simulink model "Kimura_simulink"  (R2022b)
settings: Solver=ode45  StartTime=0.0  StopTime=10  RelTol=1e-3  AbsTol=1e-6
settings Model: Creator=MSC Software  LastModifiedBy=Administrator
settings SolverCC: AutoScaleAbsTol=off  AlgebraicLoopSolver=TrustRegion
settings DataIOCC: SaveFormat=Array  SignalLoggingSaveFormat=ModelDataLogs  ReturnWorkspaceOutputs=off
settings OptimizationCC: BlockReduction=off  BooleanDataType=off  ExpressionDepthLimit=2147483647  InitFltsAndDblsToZero=on  LifeSpan=inf
settings DebuggingCC: SaveWithParameterizedLinksMsg=none  UnderspecifiedInitializationDetection=Classic  MergeDetectMultiDrivingBlocksExec=none  SignalResolutionControl=TryResolveAllWithWarning  MultiTaskDSMMsg=warning  MultiTaskCondExecSysMsg=none  FcnCallInpInsideContextMsg=warning  UnconnectedInputMsg=warning  UnconnectedOutputMsg=warning  UnconnectedLineMsg=warning  StateNameClashWarn=warning  SFUnexpectedBacktrackingDiag=warning  SFNoUnconditionalDefaultTransitionDiag=warning  SFExecutionAtInitializationDiag=none  SFMachineParentedDataDiag=warning  ArithmeticOperatorsInVariantConditions=warning
settings HardwareCC: ProdBitPerPointer=32  ProdBitPerSizeT=32  ProdBitPerPtrDiffT=32  ProdLargestAtomicFloat=None  ProdIntDivRoundTo=Undefined  ProdEndianess=Unspecified  ProdWordSize=32  ProdHWDeviceType=32-bit Generic  TargetUnknown=on
settings ModelReferenceCC: EnableRefExpFcnMdlSchedulingChecks=on  PropagateSignalLabelsOutOfModel=off
settings SFSimCC: SimUseLocalCustomCode=off  CustomCodeUndefinedFunction=UseInterfaceOnly
settings RTWCC: TemplateMakefile=grt_unix.tmf  RTWUseLocalCustomCode=off
settings CodeAppCC: StateflowObjectComments=on
settings GRTTargetCC: TargetFcnLib=ansi_tfl_tmw.mat  TargetLangStandard=C89/C90 (ANSI)  CombineOutputUpdateFcns=off  GRTInterface=on
settings ConfigComp: CovMetricSettings=dw  CovSaveCumulativeToWorkspaceVar=on  CovSaveSingleToWorkspaceVar=on  CovExternalEMLEnable=off

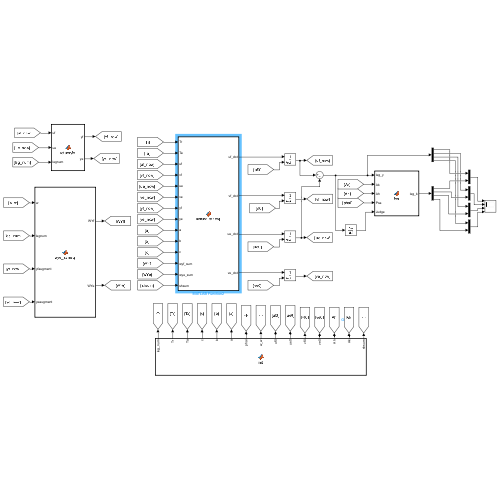
[thumbnail: Simulink's stored preview of the top-level diagram]
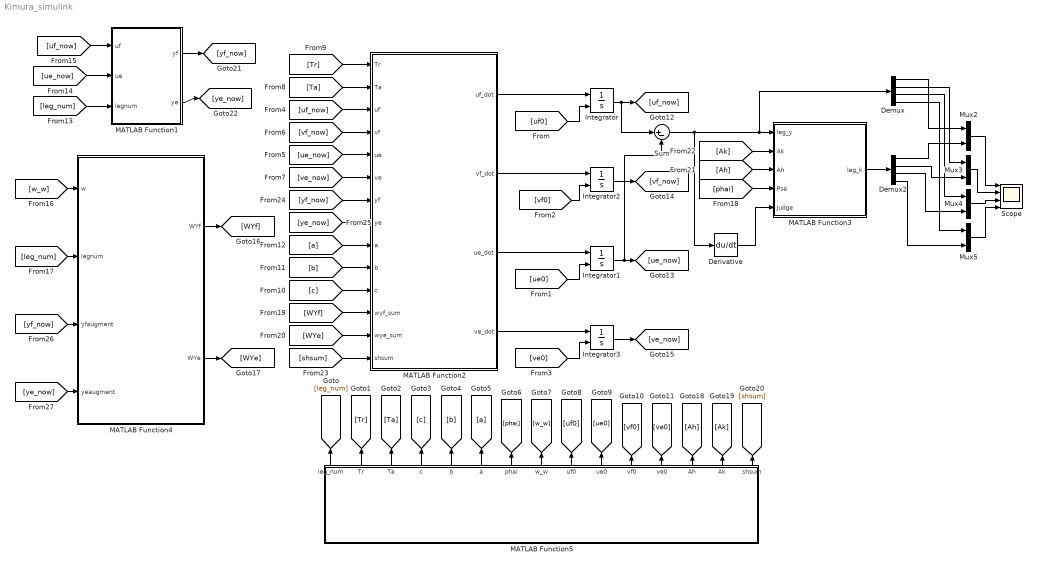
== system Kimura_simulink ==
  Demux : Demux
  Demux2 : Demux
  Derivative : Derivative
  Integrator{,1..3} (4 alike) : Integrator  InitialConditionSource=external
  MATLAB Function1 : MATLAB Function  TreatAsAtomicUnit=on
  MATLAB Function2 : MATLAB Function  TreatAsAtomicUnit=on
  MATLAB Function3 : MATLAB Function  TreatAsAtomicUnit=on
  MATLAB Function4 : MATLAB Function  TreatAsAtomicUnit=on
  MATLAB Function5 : MATLAB Function  TreatAsAtomicUnit=on
  Mux{2..5} (4 alike) : Mux  Inputs=2
  Scope : Scope  NumInputPorts=4
  Sum : Sum  Inputs=|+-
  wires:
  MATLAB Function2/4(ve_dot) -> Integrator3/1
  Demux/1 -> Mux2/1
  Mux5/1 -> Scope/4
  Demux/2 -> Mux3/1
  Demux/3 -> Mux4/1
  Mux4/1 -> Scope/3
  Demux2/3 -> Mux4/2
  Demux2/4 -> Mux5/2
  Demux2/1 -> Mux2/2
  Mux2/1 -> Scope/1
  Mux3/1 -> Scope/2
  MATLAB Function2/1(uf_dot) -> Integrator/1
  Demux2/2 -> Mux3/2
  Demux/4 -> Mux5/1
  MATLAB Function3/1(leg_k) -> Demux2/1
  MATLAB Function5/1(leg_num) -> [leg_num]
  MATLAB Function5/2(Tr) -> [Tr]
  MATLAB Function5/3(Ta) -> [Ta]
  MATLAB Function5/4(c) -> [c]
  MATLAB Function5/5(b) -> [b]
  MATLAB Function5/6(a) -> [a]
  MATLAB Function5/7(phai) -> [phai]
  MATLAB Function5/8(w_w) -> [w_w]
  MATLAB Function5/9(uf0) -> [uf0]
  MATLAB Function5/12(ve0) -> [ve0]
  MATLAB Function5/11(vf0) -> [vf0]
  MATLAB Function5/10(ue0) -> [ue0]
  [uf0] -> Integrator/2
  [ve0] -> Integrator3/2
  Integrator/1 -> Sum/1, [uf_now]
  Integrator3/1 -> [ve_now]
  [ve_now] -> MATLAB Function2/6(ve)
  [vf_now] -> MATLAB Function2/4(vf)
  [ue_now] -> MATLAB Function2/5(ue)
  [uf_now] -> MATLAB Function2/3(uf)
  [Tr] -> MATLAB Function2/1(Tr)
  [Ta] -> MATLAB Function2/2(Ta)
  [c] -> MATLAB Function2/11(c)
  [b] -> MATLAB Function2/10(b)
  [a] -> MATLAB Function2/9(a)
  [leg_num] -> MATLAB Function1/3(legnum)
  [ue_now] -> MATLAB Function1/2(ue)
  [uf_now] -> MATLAB Function1/1(uf)
  [w_w] -> MATLAB Function4/1(w)
  [leg_num] -> MATLAB Function4/2(legnum)
  [phai] -> MATLAB Function3/4(Psa)
  Sum/1 -> Derivative/1, Demux/1, MATLAB Function3/1(leg_y)
  MATLAB Function4/1(WYf) -> [WYf]
  MATLAB Function4/2(WYe) -> [WYe]
  [WYf] -> MATLAB Function2/12(wyf_sum)
  [WYe] -> MATLAB Function2/13(wye_sum)
  MATLAB Function5/13(Ah) -> [Ah]
  MATLAB Function5/14(Ak) -> [Ak]
  [Ah] -> MATLAB Function3/3(Ah)
  [Ak] -> MATLAB Function3/2(Ak)
  MATLAB Function5/15(shsum) -> [shsum]
  [shsum] -> MATLAB Function2/14(shsum)
  [yf_now] -> MATLAB Function2/7(yf)
  [ye_now] -> MATLAB Function2/8(ye)
  MATLAB Function1/1(yf) -> [yf_now]
  MATLAB Function1/2(ye) -> [ye_now]
  [yf_now] -> MATLAB Function4/3(yfaugment)
  [ye_now] -> MATLAB Function4/4(yeaugment)
  MATLAB Function2/2(vf_dot) -> Integrator2/1
  [vf0] -> Integrator2/2
  Integrator2/1 -> [vf_now]
  MATLAB Function2/3(ue_dot) -> Integrator1/1
  [ue0] -> Integrator1/2
  Integrator1/1 -> Sum/2, [ue_now]
  Derivative/1 -> MATLAB Function3/5(Judge)

== matlab function Kimura_simulink/MATLAB Function1 ==
  data: uf input; ue input; legnum input; yf output; ye output
function [yf, ye] = returnyfe(uf, ue,legnum)
    yf = zeros(4,1);
    ye= zeros(4, 1);
    for i= 1:1:legnum
        yf(i) = max(uf(i), 0);
        ye(i) = max(ue(i), 0);
    end
end

== matlab function Kimura_simulink/MATLAB Function3 ==
  data: leg_y input; leg_k output; Ak input; Ah input; Psa input; Judge input
function leg_k = fcn(leg_y,Ak,Ah,Psa,Judge)
%#codegen
thetah = 1.72071210380880;	
leg_k = zeros(4,1);
for i = 1:1:4
    if Judge(i)>0
       leg_k(i)=1*(Ak/Ah)*(1-(leg_y(i)/thetah)^2);
    else
       leg_k(i)=0;
    end
end
end

== matlab function Kimura_simulink/MATLAB Function4 ==
  data: w input; legnum input; yfaugment input; WYf output; yeaugment input; WYe output
function [WYf, WYe] = wye_sumeq(w, legnum,  yfaugment, yeaugment)
WYf= zeros(4,1);
WYe= zeros(4,1);
for i_i =1:1:legnum
    for j_j=1:1:legnum
        WYf(i_i)=WYf(i_i)+w(i_i, j_j)*yfaugment( j_j);
        WYe(i_i)=WYe(i_i)+w(i_i, j_j)*yeaugment( j_j);
    end
end

== matlab function Kimura_simulink/MATLAB Function5 ==
  data: leg_num output; Tr output; Ta output; c output; b output; a output; phai output; w_w output; uf0 output; ue0 output; vf0 output; ve0 output; Ah output; Ak output; shsum output
function [leg_num, Tr, Ta,c,b,a, phai,w_w,uf0, ue0, vf0, ve0, Ah, Ak, shsum] = init()
    leg_num=4;%足的个数
    mm=8;%m项反馈信息
    Tr=0.04;%上升时间参数
    Ta=0.38;
    c=0.23;%直流输入
    b=-2.0;%适应系数
    a=-1.0;%抑制系数
    phai=1;
    %%
    gait=2;
    w_w=zeros(leg_num,leg_num);%定义步态矩阵
    switch(gait)
        case 1
           w_w=[0 -1 1 -1;-1 0 -1 1;1 -1 0 -1;-1 1 -1 0];
        case 2
            w_w=[0 -1 -1 1;-1 0 1 -1;-1 1 0 -1;1 -1 -1 0];
        case 3
            w_w=[0 1 -1 -1;1 0 -1 -1;-1 1 0 -1;-1 -1 1 0];
        case 4
            w_w=[0 -1 -1 -1;-1 0 -1 -1;-1 -1 0 -1;-1 -1 -1 0];
        otherwise
            w_w=[0 -1 1 -1;-1 0 -1 1;1 -1 0 -1;-1 1 -1 0];   
    end
    %%
    vf=zeros(leg_num,1);
    ve=zeros(leg_num,1);
    Vfe=[vf,ve];
    %%
    yf=zeros(leg_num,1);
    ye=zeros(leg_num,1);
    Yfe=[yf,ye];
    Yef=[ye,yf];
    Y=zeros(leg_num,1);%输出的关节映射矩阵
    %%
    uf=rand(leg_num,1)*c/10;
    ue=rand(leg_num,1)*c/10;
    Ufe=[uf,ue];
    %%
    hf=zeros(mm,1);
    he=zeros(mm,1);
    Hfe=[hf,he];
    %%
    ss=zeros(leg_num,mm);
    WYf=zeros(leg_num,1);
    WYe=zeros(leg_num,1);
    SHf=zeros(leg_num,1);
    SHe=zeros(leg_num,1);
    %%
    E=zeros(leg_num,2);
    for i=1:1:leg_num
        E(i,1)=1;
        E(i,2)=1;
    end
    %% 关节参数，此处参数需实测，试验数据参考书
    h=0.02;  %抬腿高度
    v=1;   %行走速度
    T=0.4; %步态周期
    S=v*T; %步长
    l=0.4;   %腿节长度
    theta0=30/180*pi;%髋关节和膝关节平衡位置与垂直线夹角 
    L=2*l*cos(theta0);%髋关节与足端之间长度
    Ah=8.3;%asin((Beta*S)/(2*L));%髋关节摆动幅度
    Ak=5.3;%acos((l*cos(theta0)-h)/l)-theta0;%膝关节摆动幅度
    %% 时间，分辨率设置
    %对时间进行算法积分
    u0=[0.009 0.0021 0.0134 0.0022;
           0.0272 0.0003 0.0206 0.0057;
           0.0199 0.0067 0.0171 0.0111;
           0.0022 0.0151 0.0149 0.0081;];%初值会影响相序
    n=2000;
    Foot_end_x=zeros(n);%足端
    Foot_end_y=zeros(n);
    t_total = 8*pi/2;
    t=linspace(0,t_total,n);%转一圈
    ts=t_total/n;
     shsum = zeros(leg_num,1);
    % 积分计算
     uf0 = u0(:,1);
     vf0 = u0(:,2);
     ue0 = u0(:,3);
    ve0 = u0(:,4);
    shsum = zeros(leg_num,1);
end

== matlab function Kimura_simulink/MATLAB Function2 ==
  data: Tr input; Ta input; uf input; uf_dot output; vf input; ue input; ve input; yf input; vf_dot output; ye input; a input; b input; c input; wyf_sum input; wye_sum input; shsum input; ue_dot output; ve_dot output
function [uf_dot, vf_dot,ue_dot, ve_dot] = kimura_stateq(Tr, Ta, uf, vf, ue, ve, yf, ye,a, b, c,wyf_sum, wye_sum, shsum)
    uf_dot = zeros(4, 1);
    ue_dot = zeros(4, 1);
    vf_dot = zeros(4, 1);
    ve_dot = zeros(4, 1);
    uf_dot =(1/Tr)*(-uf+b*vf+a*ye+wyf_sum+shsum+c);
    vf_dot = (1/Ta)*(yf-vf);
    ue_dot = (1/Tr)*(-ue+b*ve+a*yf+wye_sum+shsum+c);
    ve_dot =  (1/Ta)*(ye-ve);
end
